simulink model "prelab"  (R2014a)
settings: Solver=ode45  StartTime=0.0  StopTime=10.0  RelTol=1e-3
settings Model: Creator=Shiyu  LastModifiedBy=Shiyu

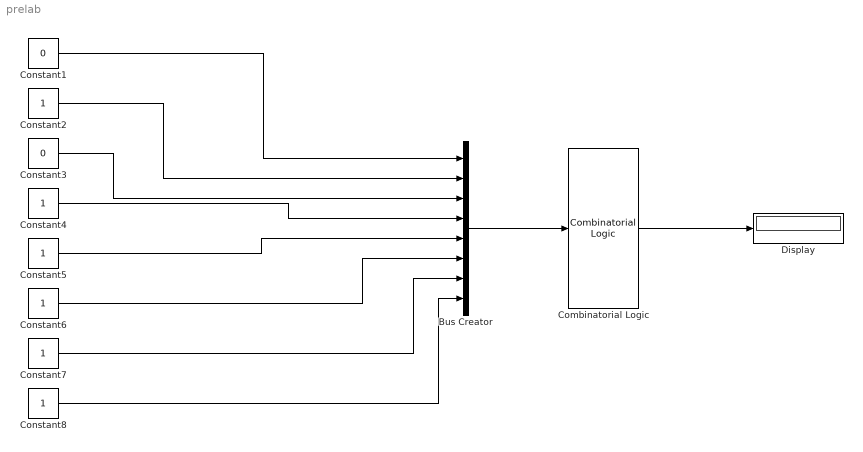
== system prelab ==
  Bus Creator : BusCreator  Inputs=8
  Combinatorial Logic : CombinatorialLogic  TruthTable=[0;1;0;1;0;1;0;0]
  Constant1 : Constant  Value=0  OutDataTypeStr=boolean
  Constant{2,4..8} (6 alike) : Constant  OutDataTypeStr=boolean
  Constant3 : Constant  Value=0  OutDataTypeStr=boolean
  Display : Display
  wires:
  Constant1/1 -> Bus Creator/1
  Constant2/1 -> Bus Creator/2
  Constant3/1 -> Bus Creator/3
  Constant4/1 -> Bus Creator/4
  Constant5/1 -> Bus Creator/5
  Constant6/1 -> Bus Creator/6
  Constant7/1 -> Bus Creator/7
  Constant8/1 -> Bus Creator/8
  Combinatorial Logic/1 -> Display/1
  Bus Creator/1 -> Combinatorial Logic/1
